simulink model "Inverter_Simulink"  (R2018a)
settings: Solver=VariableStepAuto  StartTime=0.0  StopTime=10.0  RelTol=1e-3
libraries: powerlib x9
settings Model: Creator=jflorek2012  LastModifiedBy=jflorek2012

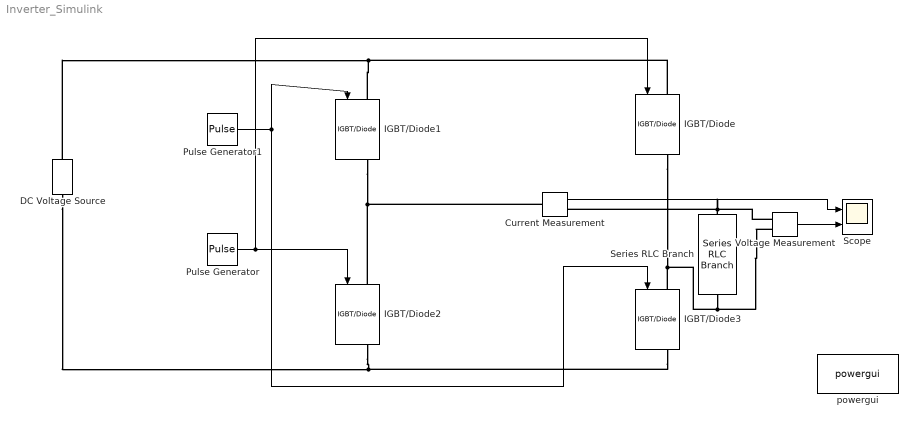
== system Inverter_Simulink ==
  Current Measurement : powerlib/Measurements/Current Measurement  PhasorSimulation=off  OutputType=Complex  PSBequivalent=0
  DC Voltage Source : powerlib/Electrical Sources/DC Voltage Source  Amplitude=12  Measurements=None
  IGBT/Diode{,1..3} (4 alike) : powerlib/Power Electronics/IGBT//Diode  Ron=1e-3  Rs=1e5  Cs=inf  Measurements=on
  Pulse Generator : DiscretePulseGenerator  PulseType=Time based  Period=10  PulseWidth=5
  Pulse Generator1 : DiscretePulseGenerator  PulseType=Time based  Period=10  PulseWidth=5  PhaseDelay=5
  Scope : Scope  NumInputPorts=2
  Series RLC Branch : powerlib/Elements/Series RLC Branch  LConnTagsString=__new0  RConnTagsString=__new0  BranchType=RLC  Resistance=1000  Inductance=.001  SetiL0=off  InitialCurrent=0  Capacitance=0  Setx0=off  InitialVoltage=0  Measurements=None
  Voltage Measurement : powerlib/Measurements/Voltage Measurement  PhasorSimulation=off  OutputType=Complex  PSBequivalent=0
  powergui : powerlib/powergui  Priority=1  SimulationMode=Continuous  SampleTime=50e-6  frequency=60  Iterations=50  frequencyindice=0  Pbase=100e6  ErrMax=1e-4  UnitsV=kV  UnitsW=MW  buscounter=0  FunctionMessages=off  echomessages=off  EnableUseOfTLC=off  CurrentSourceSwitches=off  DisableSnubberDevices=off  DisableRonSwitches=off  DisableVfSwitches=off  DisplayEquations=off  SolverType=Tustin/Backward Euler (TBE)  Interpol=off  ExternalGateDelay=off  methode=off  Ts=100  x0status=blocks  SPID=on  SwTol=0  HookPort=off  RestoreLinks=warning  ResistiveCurrentMeasurement=off  Frange=[0:2:500]  Ylog=off  Xlog=on  ShowGrid=off  save=off  variable=ZData  structure=0  ZoomFFT=off  StartTime=0.0  cycles=1  DisplayStyle=1  fundamental=60  FreqAxis=off  MaxFrequency=1000  frequencyindicesteady=1  RmsSteady=1  display=off
  wires:
  Pulse Generator1/1 -> IGBT/Diode3/1, IGBT/Diode1/1
  Pulse Generator/1 -> IGBT/Diode2/1, IGBT/Diode/1
  Current Measurement/1 -> Scope/1
  Voltage Measurement/1 -> Scope/2
  connections:
  Current Measurement/LConn1 -- IGBT/Diode1/RConn1 -- IGBT/Diode2/LConn1
  DC Voltage Source/RConn1 -- IGBT/Diode1/LConn1 -- IGBT/Diode/LConn1
  DC Voltage Source/LConn1 -- IGBT/Diode3/RConn1 -- IGBT/Diode2/RConn1
  Voltage Measurement/LConn1 -- Series RLC Branch/LConn1 -- Current Measurement/RConn1
  Voltage Measurement/LConn2 -- Series RLC Branch/RConn1 -- IGBT/Diode/RConn1 -- IGBT/Diode3/LConn1
